simulink model "ReceiveWrite"  (R2016b)
settings: Solver=FixedStepDiscrete  StartTime=0.0  StopTime=inf  FixedStep=sCoreParams.core.stepPeriod  RelTol=1e-3  EnableMultiTasking=on
values from neighbouring files (symbols this model uses):
  sCoreParams = InitCoreParams    [ClosedLoopStimConsole.m]    (also in CompileModelComplete.m; NeuroModConsole.m)
libraries: dspnetwork x8, xpcutilitieslib x3, xpcrtudplib x3
settings Model: Creator=User  LastModifiedBy=Rina
settings SolverCC: EnableConcurrentExecution=on
settings DataIOCC: SaveFormat=Array  SaveOutput=off  SignalLogging=off  DSMLogging=off  SaveTime=off
settings OptimizationCC: BlockReduction=off  DefaultParameterBehavior=Inlined  OptimizeBlockIOStorage=off  BufferReuse=off  GlobalBufferReuse=off  ExpressionFolding=off  LocalBlockOutputs=off  LifeSpan=inf
settings DebuggingCC: SolverPrmCheckMsg=warning  InheritedTsInSrcMsg=none  UnconnectedInputMsg=none  UnconnectedOutputMsg=none  UnconnectedLineMsg=none  StateNameClashWarn=warning  SFUnexpectedBacktrackingDiag=warning  SFNoUnconditionalDefaultTransitionDiag=warning  SFExecutionAtInitializationDiag=none
settings HardwareCC: ProdBitPerPointer=32  ProdBitPerSizeT=32  ProdBitPerPtrDiffT=32  ProdLargestAtomicFloat=None  ProdWordSize=32  ProdLongLongMode=on  ProdHWDeviceType=Generic->32-bit x86 compatible
settings ModelReferenceCC: ModelReferenceNumInstancesAllowed=Single  PropagateSignalLabelsOutOfModel=off
settings RTWCC: SystemTargetFile=slrt.tlc  TemplateMakefile=slrt_default_tmf  Description=Simulink Real-Time  RTWCompilerOptimization=on
settings TargetCC: CodeReplacementLibrary=XPC_BLAS  ParMdlRefBuildCompliant=on  ConcurrentExecutionCompliant=on  GeneratePreprocessorConditionals=Use local settings  MatFileLogging=on  MATLABClassNameForMDSCustomization=xpcAperiodicCustomization
settings ConfigComp: CovMetricSettings=dw  CovHtmlReporting=on  CovSaveCumulativeToWorkspaceVar=on  CovSaveSingleToWorkspaceVar=on  CovExternalEMLEnable=off

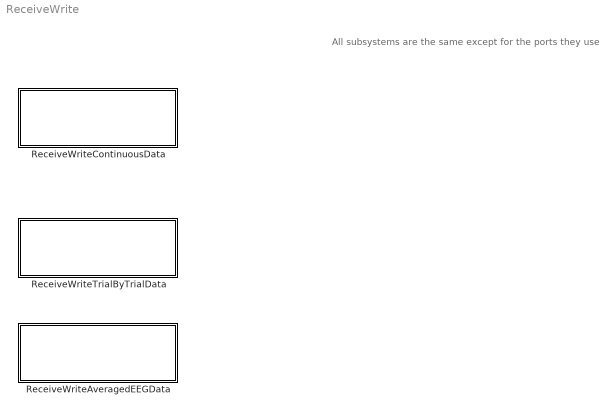
== system ReceiveWrite ==
  note: All subsystems are the same except for the ports they use
  ReceiveWriteAveragedEEGData : Subsystem
  ReceiveWriteContinuousData : Subsystem
  ReceiveWriteTrialByTrialData : Subsystem

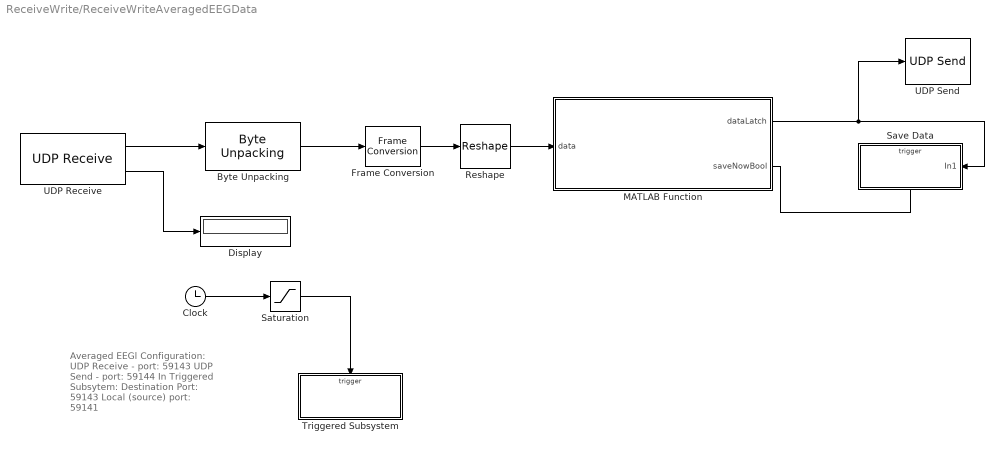
== system ReceiveWrite/ReceiveWriteAveragedEEGData ==
  note: Averaged EEGl Configuration:
      | UDP Receive - port: 59143
      | UDP Send - port: 59144
      |
      | In Triggered Subsytem:
      | Destination Port: 59143
      | Local (source) port: 59141
  "Byte Unpacking " : xpcutilitieslib/Byte Unpacking   MaskUnpackedDataTypes={'double'}  MaskUnpackedDataSizes={[sCoreParams.write.maxAveragedDataPerStep*sCoreParams.write.broadcastAvEEGSamp]}  MaskAlignment=1
  Clock : Clock
  Display : Display
  Frame Conversion : FrameConversion  InheritSamplingMode=off  OutFrame=Sample-based
  MATLAB Function : MATLAB Function  TreatAsAtomicUnit=on
  Reshape : Reshape  OutputDimensionality=Customize  OutputDimensions=[sCoreParams.write.maxAveragedDataPerStep, sCoreParams.write.broadcastAvEEGSamp]
  Saturation : Saturate  UpperLimit=.05  LowerLimit=0
  Save Data : Subsystem
  Triggered Subsystem : Subsystem  TreatAsAtomicUnit=on
  UDP Receive : dspnetwork/UDP Receive  localURL='0.0.0.0'  localPort=59143  remoteURL='0.0.0.0'  remotePort=-1  recvBufferSize=8192*8  dims=sCoreParams.write.maxAveragedDataPerStep*sCoreParams.write.broadcastAvEEGSamp*8  signalDatatype=uint8  isVarSize=off  showBlockingTime=off  blockingTime=0  sampletime=-1
  UDP Send : dspnetwork/UDP Send  remoteURL='127.0.0.1'  remotePort=59144  localURL='0.0.0.0'  localPortSource=Automatically determine  localPort=-1  sampletime=-1  separateLengthPort=0
  wires:
  "Byte Unpacking "/1 -> Frame Conversion/1
  UDP Receive/1 -> "Byte Unpacking "/1
  MATLAB Function/1(dataLatch) -> UDP Send/1, Save Data/1(In1)
  Clock/1 -> Saturation/1
  Saturation/1 -> Triggered Subsystem/Trigger
  Frame Conversion/1 -> Reshape/1
  Reshape/1 -> MATLAB Function/1(data)
  MATLAB Function/2(saveNowBool) -> Save Data/Trigger
  UDP Receive/2 -> Display/1

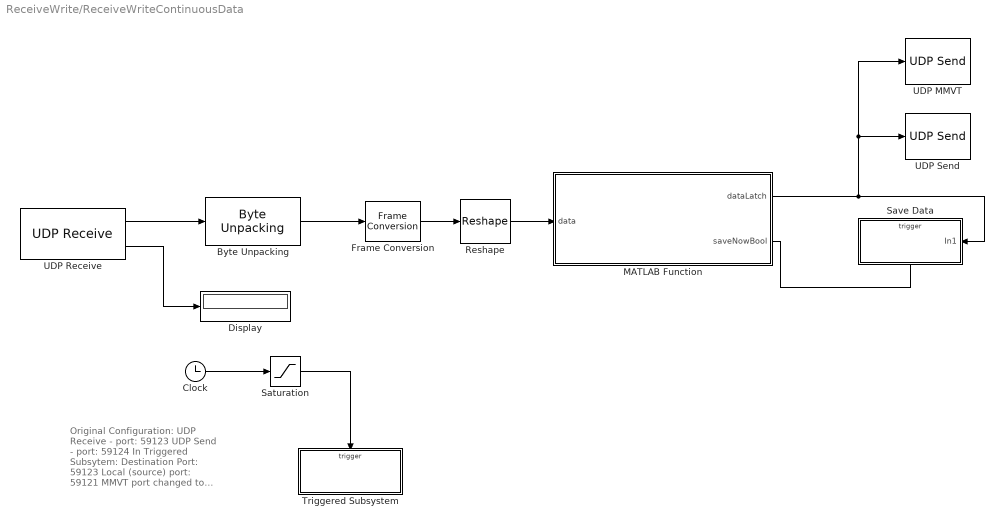
== system ReceiveWrite/ReceiveWriteContinuousData ==
  note: Original Configuration:
      | UDP Receive - port: 59123
      | UDP Send - port: 59124
      |
      | In Triggered Subsytem:
      | Destination Port: 59123
      | Local (source) port: 59121
      |
      | MMVT port changed to 59164
  "Byte Unpacking " : xpcutilitieslib/Byte Unpacking   MaskUnpackedDataTypes={'double'}  MaskUnpackedDataSizes={[sCoreParams.write.maxContinuousSignalsPerStep*sCoreParams.write.broadcastSamp]}  MaskAlignment=1
  Clock : Clock
  Display : Display
  Frame Conversion : FrameConversion  InheritSamplingMode=off  OutFrame=Sample-based
  MATLAB Function : MATLAB Function  TreatAsAtomicUnit=on
  Reshape : Reshape  OutputDimensionality=Customize  OutputDimensions=[sCoreParams.write.broadcastSamp,sCoreParams.write.maxContinuousSignalsPerStep]
  Saturation : Saturate  UpperLimit=.05  LowerLimit=0
  Save Data : Subsystem
  Triggered Subsystem : Subsystem  TreatAsAtomicUnit=on
  UDP MMVT : dspnetwork/UDP Send  remoteURL='127.0.0.1'  remotePort=59164  localURL='0.0.0.0'  localPortSource=Automatically determine  localPort=-1  sampletime=-1  separateLengthPort=0
  UDP Receive : dspnetwork/UDP Receive  localURL='0.0.0.0'  localPort=59123  remoteURL='0.0.0.0'  remotePort=-1  recvBufferSize=8192*8  dims=sCoreParams.write.maxContinuousSignalsPerStep*sCoreParams.write.broadcastSamp*8  signalDatatype=uint8  isVarSize=off  showBlockingTime=off  blockingTime=0  sampletime=-1
  UDP Send : dspnetwork/UDP Send  remoteURL='127.0.0.1'  remotePort=59124  localURL='0.0.0.0'  localPortSource=Automatically determine  localPort=-1  sampletime=-1  separateLengthPort=0
  wires:
  "Byte Unpacking "/1 -> Frame Conversion/1
  UDP Receive/1 -> "Byte Unpacking "/1
  MATLAB Function/1(dataLatch) -> UDP MMVT/1, UDP Send/1, Save Data/1(In1)
  Clock/1 -> Saturation/1
  Saturation/1 -> Triggered Subsystem/Trigger
  Frame Conversion/1 -> Reshape/1
  Reshape/1 -> MATLAB Function/1(data)
  MATLAB Function/2(saveNowBool) -> Save Data/Trigger
  UDP Receive/2 -> Display/1

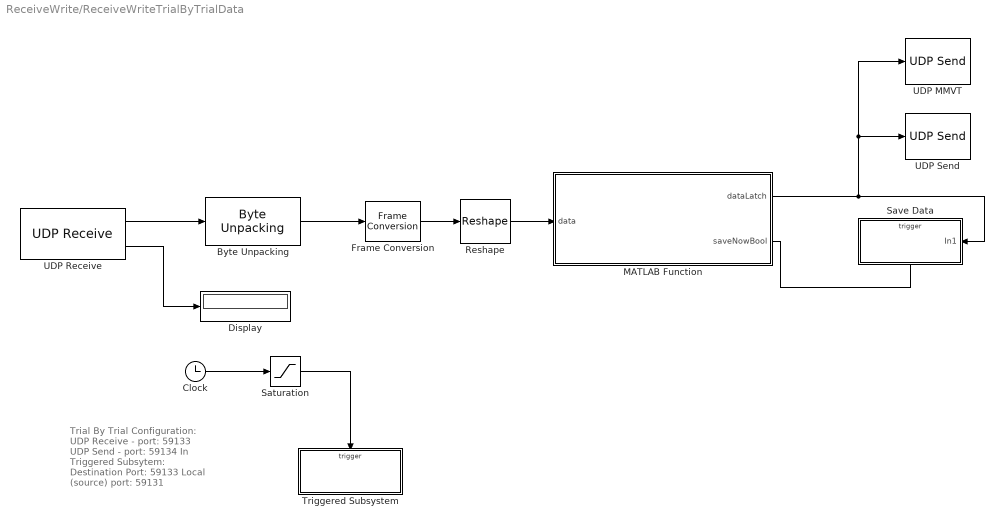
== system ReceiveWrite/ReceiveWriteTrialByTrialData ==
  note: Trial By Trial Configuration:
      | UDP Receive - port: 59133
      | UDP Send - port: 59134
      |
      | In Triggered Subsytem:
      | Destination Port: 59133
      | Local (source) port: 59131
  "Byte Unpacking " : xpcutilitieslib/Byte Unpacking   MaskUnpackedDataTypes={'double'}  MaskUnpackedDataSizes={[sCoreParams.write.maxTrialByTrialDataPerStep]}  MaskAlignment=1
  Clock : Clock
  Display : Display
  Frame Conversion : FrameConversion  InheritSamplingMode=off  OutFrame=Sample-based
  MATLAB Function : MATLAB Function  TreatAsAtomicUnit=on
  Reshape : Reshape  OutputDimensionality=Customize  OutputDimensions=[1,sCoreParams.write.maxTrialByTrialDataPerStep]
  Saturation : Saturate  UpperLimit=.05  LowerLimit=0
  Save Data : Subsystem
  Triggered Subsystem : Subsystem  TreatAsAtomicUnit=on
  UDP MMVT : dspnetwork/UDP Send  remoteURL='127.0.0.1'  remotePort=59154  localURL='0.0.0.0'  localPortSource=Automatically determine  localPort=-1  sampletime=-1  separateLengthPort=0
  UDP Receive : dspnetwork/UDP Receive  localURL='0.0.0.0'  localPort=59133  remoteURL='0.0.0.0'  remotePort=-1  recvBufferSize=8192*8  dims=sCoreParams.write.maxTrialByTrialDataPerStep*8  signalDatatype=uint8  isVarSize=off  showBlockingTime=off  blockingTime=0  sampletime=-1
  UDP Send : dspnetwork/UDP Send  remoteURL='127.0.0.1'  remotePort=59134  localURL='0.0.0.0'  localPortSource=Automatically determine  localPort=-1  sampletime=-1  separateLengthPort=0
  wires:
  "Byte Unpacking "/1 -> Frame Conversion/1
  UDP Receive/1 -> "Byte Unpacking "/1
  MATLAB Function/1(dataLatch) -> UDP MMVT/1, UDP Send/1, Save Data/1(In1)
  Clock/1 -> Saturation/1
  Saturation/1 -> Triggered Subsystem/Trigger
  Frame Conversion/1 -> Reshape/1
  Reshape/1 -> MATLAB Function/1(data)
  MATLAB Function/2(saveNowBool) -> Save Data/Trigger
  UDP Receive/2 -> Display/1

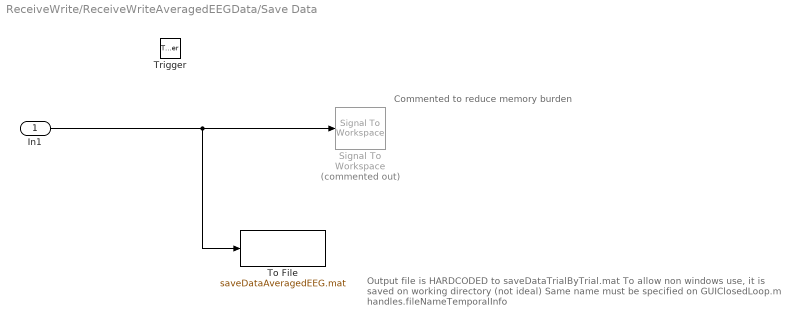
== system ReceiveWrite/ReceiveWriteAveragedEEGData/Save Data ==
  note: Commented to reduce memory burden
  note: Output file is HARDCODED to saveDataTrialByTrial.mat
      | To allow non windows use, it is saved on working directory (not ideal)
      | Same name must be specified on GUIClosedLoop.m handles.fileNameTemporalInfo
  In1 : Inport
  Trigger : TriggerPort  VariantControl=Variant
  Signal To Workspace : SignalToWorkspace  Commented=on  VariableName=savedData
      settings: CopyFcn=dspblkcopystw(gcbh);
  "To File " : ToFile  Filename=saveDataAveragedEEG.mat  MatrixName=savedDataAveragedEEG  SaveFormat=Timeseries
  wires:
  In1/1 -> "To File "/1, Signal To Workspace/1

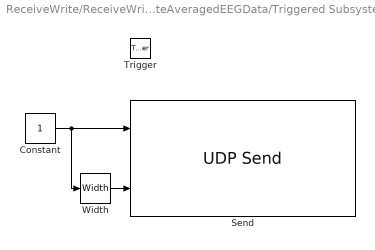
== system ReceiveWrite/ReceiveWriteAveragedEEGData/Triggered Subsystem ==
  Trigger : TriggerPort  TriggerType=either  VariantControl=Variant
  Constant : Constant  OutDataTypeStr=uint8
  Send : xpcrtudplib/UDP Send  ipAddressVal=Use host-target connection  localPort=59141  toAddress=255.255.255.255  toPort=59143  sampleTime=-1
  Width : Width
  wires:
  Constant/1 -> Width/1, Send/1
  Width/1 -> Send/2

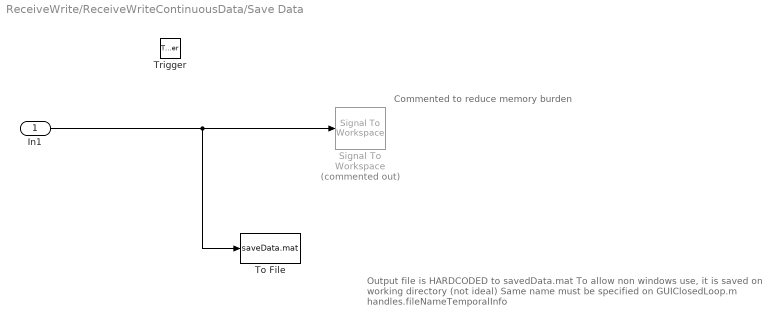
== system ReceiveWrite/ReceiveWriteContinuousData/Save Data ==
  note: Commented to reduce memory burden
  note: Output file is HARDCODED to savedData.mat
      | To allow non windows use, it is saved on working directory (not ideal)
      | Same name must be specified on GUIClosedLoop.m handles.fileNameTemporalInfo
  In1 : Inport
  Trigger : TriggerPort  VariantControl=Variant
  Signal To Workspace : SignalToWorkspace  Commented=on  VariableName=savedData
      settings: CopyFcn=dspblkcopystw(gcbh);
  "To File " : ToFile  Filename=saveData.mat  MatrixName=savedData  SaveFormat=Timeseries
  wires:
  In1/1 -> "To File "/1, Signal To Workspace/1

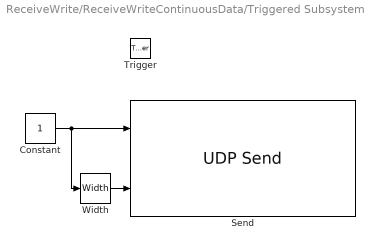
== system ReceiveWrite/ReceiveWriteContinuousData/Triggered Subsystem ==
  Trigger : TriggerPort  TriggerType=either  VariantControl=Variant
  Constant : Constant  OutDataTypeStr=uint8
  Send : xpcrtudplib/UDP Send  ipAddressVal=Use host-target connection  localPort=59121  toAddress=255.255.255.255  toPort=59123  sampleTime=-1
  Width : Width
  wires:
  Constant/1 -> Width/1, Send/1
  Width/1 -> Send/2

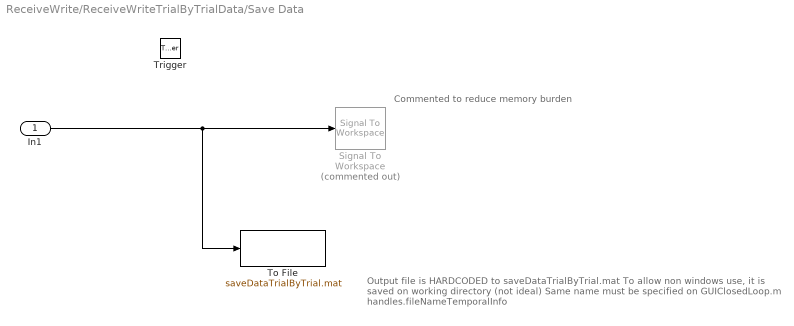
== system ReceiveWrite/ReceiveWriteTrialByTrialData/Save Data ==
  note: Commented to reduce memory burden
  note: Output file is HARDCODED to saveDataTrialByTrial.mat
      | To allow non windows use, it is saved on working directory (not ideal)
      | Same name must be specified on GUIClosedLoop.m handles.fileNameTemporalInfo
  In1 : Inport
  Trigger : TriggerPort  VariantControl=Variant
  Signal To Workspace : SignalToWorkspace  Commented=on  VariableName=savedData
      settings: CopyFcn=dspblkcopystw(gcbh);
  "To File " : ToFile  Filename=saveDataTrialByTrial.mat  MatrixName=savedDataTrialByTrial  SaveFormat=Timeseries
  wires:
  In1/1 -> "To File "/1, Signal To Workspace/1

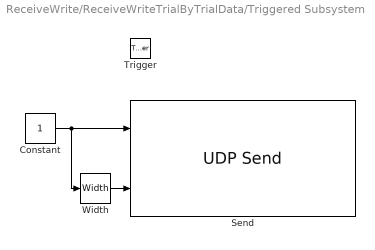
== system ReceiveWrite/ReceiveWriteTrialByTrialData/Triggered Subsystem ==
  Trigger : TriggerPort  TriggerType=either  VariantControl=Variant
  Constant : Constant  OutDataTypeStr=uint8
  Send : xpcrtudplib/UDP Send  ipAddressVal=Use host-target connection  localPort=59131  toAddress=255.255.255.255  toPort=59133  sampleTime=-1
  Width : Width
  wires:
  Constant/1 -> Width/1, Send/1
  Width/1 -> Send/2

== matlab function ReceiveWrite/ReceiveWriteTrialByTrialData/MATLAB Function ==
  data: data input; dataLatch output; saveNowBool output
function [dataLatch,saveNowBool] = latchData(data)
%#codegen

persistent dataPrev tsPrev

if isempty(dataPrev)
    dataPrev = zeros(size(data),class(data));
    tsPrev = 0;
end

saveNowBool = false;

if ~isequal(dataPrev,data) && any(any(data));
    dataPrev = data;
    saveNowBool = true;
    ts = dataPrev(1);
    if ts ~= (tsPrev+1)
        % Yikes!
    end
    tsPrev = ts;
end
dataLatch = dataPrev;

== matlab function ReceiveWrite/ReceiveWriteContinuousData/MATLAB Function ==
  data: data input; dataLatch output; saveNowBool output
function [dataLatch,saveNowBool] = latchData(data)
%#codegen

persistent dataPrev tsPrev

if isempty(dataPrev)
    dataPrev = zeros(size(data),class(data));
    tsPrev = 0;
end

saveNowBool = false;

if ~isequal(dataPrev,data) && any(any(data));
    dataPrev = data;
    saveNowBool = true;
    ts = dataPrev(1);
    if ts ~= (tsPrev+1)
        % Yikes!
    end
    tsPrev = ts;
end
dataLatch = dataPrev;

== matlab function ReceiveWrite/ReceiveWriteAveragedEEGData/MATLAB Function ==
  data: data input; dataLatch output; saveNowBool output
function [dataLatch,saveNowBool] = latchData(data)
%#codegen

persistent dataPrev tsPrev

if isempty(dataPrev)
    dataPrev = zeros(size(data),class(data));
    tsPrev = 0;
end

saveNowBool = false;

if ~isequal(dataPrev,data) && any(any(data));
    dataPrev = data;
    saveNowBool = true;
    ts = dataPrev(1);
    if ts ~= (tsPrev+1)
        % Yikes!
    end
    tsPrev = ts;
end
dataLatch = dataPrev;
